simulink model "es_motore_con_controllo_velocita"  (Simulink 3.00)
settings: Solver=ode45  StartTime=0.0  StopTime=60.0  RelTol=1e-6
values from neighbouring files (symbols this model uses):
  Kc = 0.1    [es_motore_fdt.m]
libraries: cstblocks x2

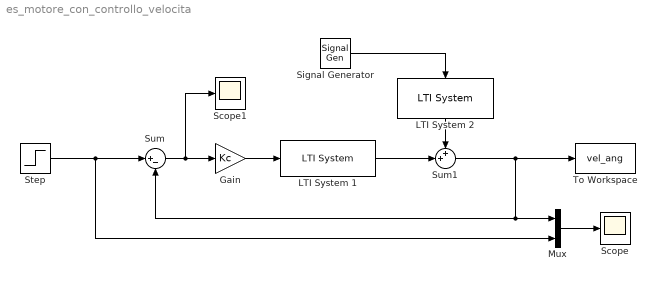
== system es_motore_con_controllo_velocita ==
  Gain : Gain  Gain=Kc  SaturateOnIntegerOverflow=off
  LTI System 1 : cstblocks/LTI System  sys=F1  IC=[0]
  LTI System 2 : cstblocks/LTI System  Orientation=down  sys=F2  IC=[0]
  Mux : Mux  Inputs=2
  Scope : Scope
      settings: TimeRange=auto  YMin=-5  YMax=5  SaveToWorkspace=off  SaveName=ScopeData
  Scope1 : Scope
      settings: TimeRange=auto  YMin=-5  YMax=5  SaveToWorkspace=off  SaveName=ScopeData
  Signal Generator : SignalGenerator  WaveForm=square  Amplitude=0.05  Frequency=0.1  Units=Hertz
  Step : Step  Time=0  Before=0  After=1  SampleTime=0
  Sum : Sum  Inputs=|+-  SaturateOnIntegerOverflow=on
  Sum1 : Sum  Inputs=++|  SaturateOnIntegerOverflow=on
  To Workspace : ToWorkspace  VariableName=vel_ang  SampleTime=-1  SaveFormat=Matrix
  wires:
  Step/1 -> Sum/1, Mux/2
  Mux/1 -> Scope/1
  Gain/1 -> LTI System 1/1
  LTI System 1/1 -> Sum1/2
  LTI System 2/1 -> Sum1/1
  Sum1/1 -> To Workspace/1, Sum/2, Mux/1
  Signal Generator/1 -> LTI System 2/1
  Sum/1 -> Gain/1, Scope1/1
